simulink model "parte3_DC1A_0214"  (R2019b)
settings: Solver=VariableStepAuto  StartTime=0.0  StopTime=50  RelTol=1e-3
values from neighbouring files (symbols this model uses):
  AEX = 0.014    [parte3_DC1A_data.m]    (also in parte3_eje3_EXAC1.m = 0.1; parte3_eje3_EXAC2.m = 0.1)
  BEX = 1.55    [parte3_DC1A_data.m]    (also in parte3_eje3_EXAC1.m = 0.03; parte3_eje3_EXAC2.m = 0.03)
  KA = 187    [parte3_DC1A_data.m]    (also in parte3_eje2_SMIB_Exc_graph.m = 1000; parte3_eje6_ESST1A.m = 51)
  KE = 1    [parte3_DC1A_data.m]
  KF = 0.058    [parte3_DC1A_data.m]    (also in parte3_eje6_ESST1A.m = 0.1)
  TA = 0.89    [parte3_DC1A_data.m]    (also in parte3_eje2_SMIB_Exc_graph.m = 0.1; parte3_eje6_ESST1A.m = 0.01)
  TB = 0.06    [parte3_DC1A_data.m]    (also in parte3_eje6_ESST1A.m = 10)
  TC = 0.173    [parte3_DC1A_data.m]    (also in parte3_eje6_ESST1A.m = 0.01)
  TE = 1.15    [parte3_DC1A_data.m]
  TF = 0.62    [parte3_DC1A_data.m]    (also in parte3_eje6_ESST1A.m = 0.31)
  VRMAX = 1.7    [parte3_DC1A_data.m]    (also in parte3_eje5_ESSTB.m = 1; parte3_eje6_ESST1A.m = 3.4)
  VRMIN = -1.7    [parte3_DC1A_data.m]    (also in parte3_eje5_ESSTB.m = -0.87; parte3_eje6_ESST1A.m = -3.4)
  VUEL = -0.01    [parte3_DC1A_data.m]
settings Model: Creator=cjuar  LastModifiedBy=cjuar

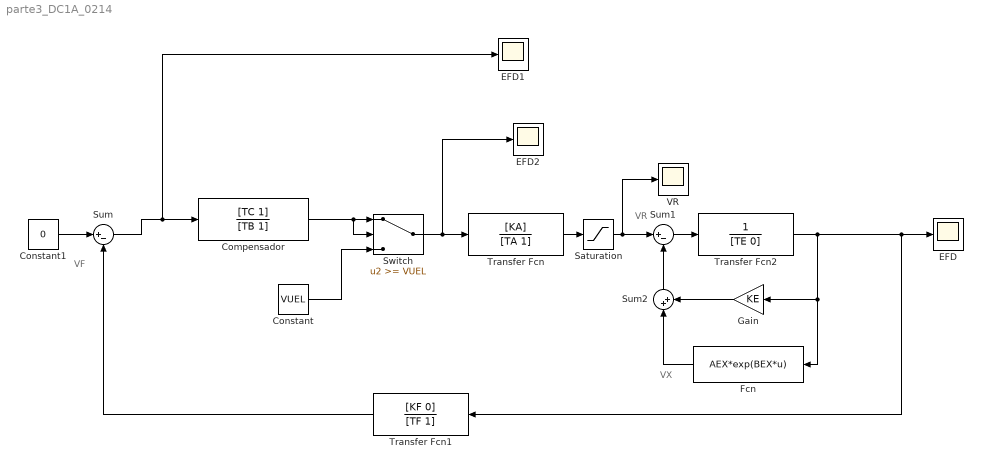
== system parte3_DC1A_0214 ==
  note: VX
  note: VR
  note: VF
  Compensador : TransferFcn  Numerator=[TC 1]  Denominator=[TB 1]
  Constant : Constant  Value=VUEL
  Constant1 : Constant  Value=0
  EFD : Scope
  EFD1 : Scope
  EFD2 : Scope
  Fcn : Fcn  Expr=AEX*exp(BEX*u)
  Gain : Gain  Gain=KE
  Saturation : Saturate  UpperLimit=VRMAX  LowerLimit=VRMIN
  Sum : Sum  Inputs=|+-
  Sum1 : Sum  Inputs=|+-
  Sum2 : Sum  Inputs=|++
  Switch : Switch  Threshold=VUEL
  Transfer Fcn : TransferFcn  Numerator=[KA]  Denominator=[TA 1]
  Transfer Fcn1 : TransferFcn  Numerator=[KF 0]  Denominator=[TF 1]
  Transfer Fcn2 : TransferFcn  Denominator=[TE 0]
  VR : Scope
  wires:
  Transfer Fcn1/1 -> Sum/2
  Sum/1 -> EFD1/1, Compensador/1
  Transfer Fcn/1 -> Saturation/1
  Saturation/1 -> VR/1, Sum1/1
  Sum1/1 -> Transfer Fcn2/1
  Gain/1 -> Sum2/2
  Sum2/1 -> Sum1/2
  Transfer Fcn2/1 -> Transfer Fcn1/1, EFD/1, Fcn/1, Gain/1
  Fcn/1 -> Sum2/1
  Compensador/1 -> Switch/1, Switch/2
  Constant/1 -> Switch/3
  Constant1/1 -> Sum/1
  Switch/1 -> EFD2/1, Transfer Fcn/1
